simulink model "prelab"  (R2022a)
settings: Solver=FixedStepAuto  StartTime=0.0  StopTime=1  FixedStep=0.001  RelTol=1e-3
values from neighbouring files (symbols this model uses):
  K = 97/5    (= 19.4)    [lab_ex2_plot.m]    (also in prelab_plot.m)
  Kd = (10*sqrt(3)-5)/388    [lab_ex2_plot.m]    (also in prelab_plot.m)
  Kr = 1+3/(5*K)    (= 1.03092783505)    [lab_ex2_plot.m]    (also in prelab_plot.m)
settings Model: Creator=zhong  LastModifiedBy=zhong

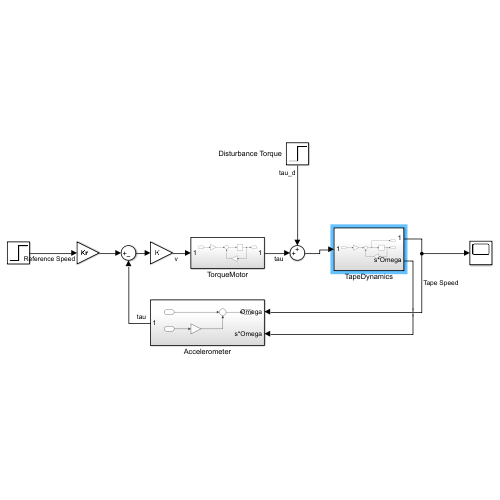
[thumbnail: Simulink's stored preview of the top-level diagram]
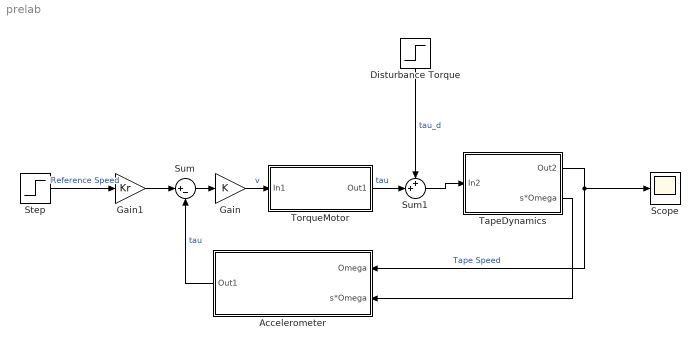
== system prelab ==
  Accelerometer : Subsystem
  Disturbance Torque : Step  Time=0  After=0  SampleTime=0
  Gain : Gain  Gain=K
  Gain1 : Gain  Gain=Kr
  Scope : Scope
  Step : Step  Time=0  SampleTime=0
  Sum : Sum  Inputs=|+-
  Sum1 : Sum  Inputs=++|
  TapeDynamics : Subsystem
  TorqueMotor : Subsystem
  wires:
  Step/1 -> Gain1/1  "Reference Speed"
  Gain1/1 -> Sum/1
  Sum/1 -> Gain/1
  Gain/1 -> TorqueMotor/1(In1)  "v"
  TorqueMotor/1(Out1) -> Sum1/2  "tau"
  Sum1/1 -> TapeDynamics/1(In2)
  TapeDynamics/1(Out2) -> Accelerometer/1(Omega), Scope/1  "Tape Speed"
  Disturbance Torque/1 -> Sum1/1  "tau_d"
  Accelerometer/1(Out1) -> Sum/2  "tau"
  TapeDynamics/2(s*Omega) -> Accelerometer/2(s*Omega)

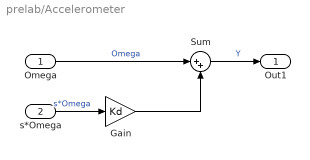
== system prelab/Accelerometer ==
  Omega : Inport
  s*Omega : Inport  Port=2
  Gain : Gain  Gain=Kd
  Sum : Sum  Inputs=|++
  Out1 : Outport
  wires:
  s*Omega/1 -> Gain/1  "s*Omega"
  Gain/1 -> Sum/2
  Omega/1 -> Sum/1  "Omega"
  Sum/1 -> Out1/1  "Y"

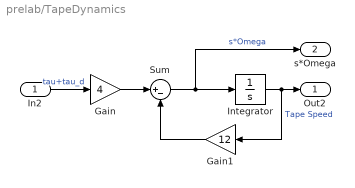
== system prelab/TapeDynamics ==
  In2 : Inport
  Gain : Gain  Gain=4
  Gain1 : Gain  Gain=12
  Integrator : Integrator
  Sum : Sum  Inputs=|+-
  Out2 : Outport
  s*Omega : Outport  Port=2
  wires:
  In2/1 -> Gain/1  "tau+tau_d"
  Gain1/1 -> Sum/2
  Gain/1 -> Sum/1
  Integrator/1 -> Gain1/1, Out2/1  "Tape Speed"
  Sum/1 -> s*Omega/1, Integrator/1  "s*Omega"

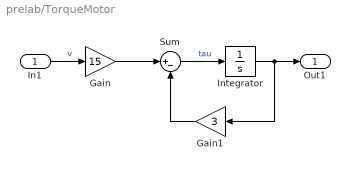
== system prelab/TorqueMotor ==
  In1 : Inport
  Gain : Gain  Gain=15
  Gain1 : Gain  Gain=3
  Integrator : Integrator
  Sum : Sum  Inputs=|+-
  Out1 : Outport
  wires:
  In1/1 -> Gain/1  "v"
  Gain/1 -> Sum/1
  Gain1/1 -> Sum/2
  Sum/1 -> Integrator/1  "tau"
  Integrator/1 -> Gain1/1, Out1/1
